simulink model "drivetrain"  (R2024a)
settings: Solver=VariableStepAuto  StartTime=0.0  StopTime=10.0  RelTol=1e-3
values from neighbouring files (symbols this model uses):
  drivetrain_gain = 10.5    [assignment_2.m]
  motor_eff = 0.9    [assignment_2.m]
  trans_eff = 0.95    [assignment_2.m]
undefined symbols (not defined in the file or in its folder): peak_m_power, peak_m_torque
settings Model: Creator=fjmo  LastModifiedBy=fjmo

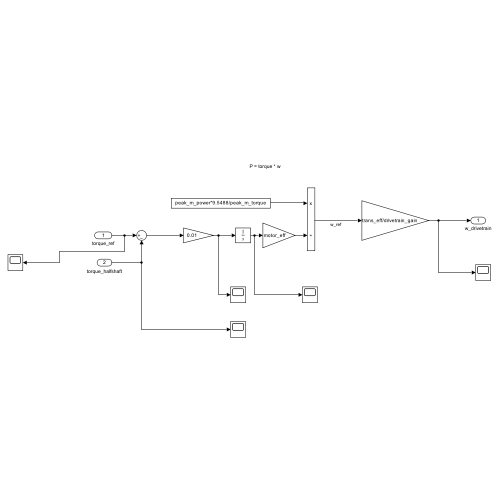
[thumbnail: Simulink's stored preview of the top-level diagram]
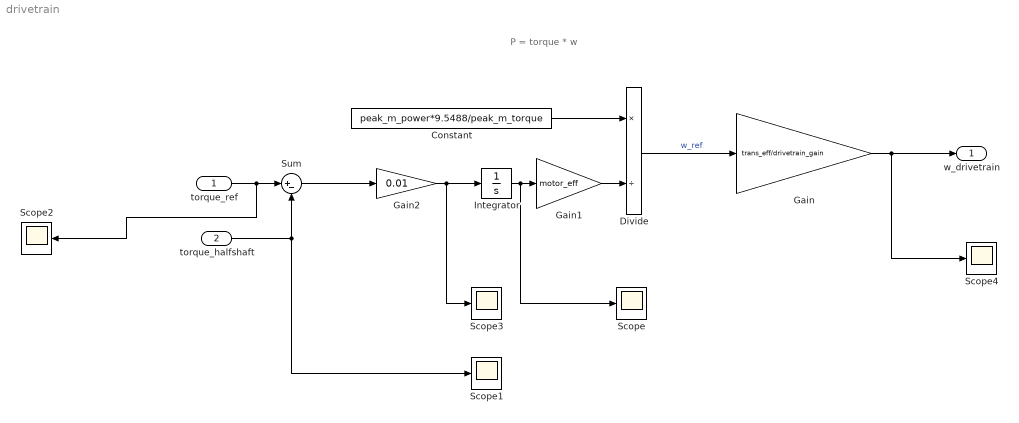
== system drivetrain ==
  note: P = torque * w
  torque_ref : Inport
  torque_halfshaft : Inport  Port=2
  Constant : Constant  Value=peak_m_power*9.5488/peak_m_torque
  Divide : Product  Inputs=*/
  Gain : Gain  Gain=trans_eff/drivetrain_gain
  Gain1 : Gain  Gain=motor_eff
  Gain2 : Gain  Gain=0.01
  Integrator : Integrator  InitialCondition=56
  Scope{,1..4} (5 alike) : Scope
  Sum : Sum  Inputs=|+-
  w_drivetrain : Outport
  wires:
  Constant/1 -> Divide/1
  Divide/1 -> Gain/1  "w_ref"
  torque_halfshaft/1 -> Sum/2, Scope1/1
  torque_ref/1 -> Scope2/1, Sum/1
  Gain/1 -> Scope4/1, w_drivetrain/1
  Gain1/1 -> Divide/2
  Integrator/1 -> Scope/1, Gain1/1
  Gain2/1 -> Scope3/1, Integrator/1
  Sum/1 -> Gain2/1
